simulink model "qss_hybrid_electric_vehicle_example"  (R2023b)
settings: Solver=VariableStepDiscrete  StartTime=0.0  StopTime=1220  RelTol=1e-3  EnableMultiTasking=on
undefined symbols (not defined in the file or in its folder): c_BT_E1, c_BT_E2, c_BT_E3, c_BT_E4, c_BT_L1, c_BT_L2, c_BT_L3, c_BT_L4, h, H_u, I_BT_max, Q_BT_0, Q_BT_IC, rho_f
libraries: qss_tb_library x5
settings Model: Creator=d_goerges  LastModifiedBy=PRATIK
settings SolverCC: AlgebraicLoopSolver=TrustRegion
settings DataIOCC: LimitDataPoints=on  SaveFormat=Array  SignalLoggingSaveFormat=ModelDataLogs  ReturnWorkspaceOutputs=off
settings OptimizationCC: ExpressionDepthLimit=2147483647  LifeSpan=inf
settings DebuggingCC: UnderspecifiedInitializationDetection=Classic  MergeDetectMultiDrivingBlocksExec=none  SolverPrmCheckMsg=warning  FcnCallInpInsideContextMsg=warning  UnconnectedInputMsg=warning  UnconnectedOutputMsg=warning  UnconnectedLineMsg=warning  StateNameClashWarn=warning  SFUnexpectedBacktrackingDiag=warning  SFNoUnconditionalDefaultTransitionDiag=warning  SFExecutionAtInitializationDiag=none  ArithmeticOperatorsInVariantConditions=warning
settings HardwareCC: ProdBitPerPointer=32  ProdBitPerSizeT=32  ProdBitPerPtrDiffT=32  ProdLargestAtomicFloat=None  ProdIntDivRoundTo=Undefined  ProdEndianess=Unspecified  ProdWordSize=32  ProdHWDeviceType=32-bit Generic
settings ModelReferenceCC: PropagateSignalLabelsOutOfModel=off
settings SFSimCC: SimUseLocalCustomCode=off  CustomCodeUndefinedFunction=UseInterfaceOnly
settings RTWCC: RTWUseLocalCustomCode=off
settings CodeAppCC: StateflowObjectComments=on
settings GRTTargetCC: TargetLangStandard=C89/C90 (ANSI)  CombineOutputUpdateFcns=off  GRTInterface=on
settings ConfigComp: CovMetricSettings=dw  CovSaveCumulativeToWorkspaceVar=on  CovSaveSingleToWorkspaceVar=on  CovExternalEMLEnable=off

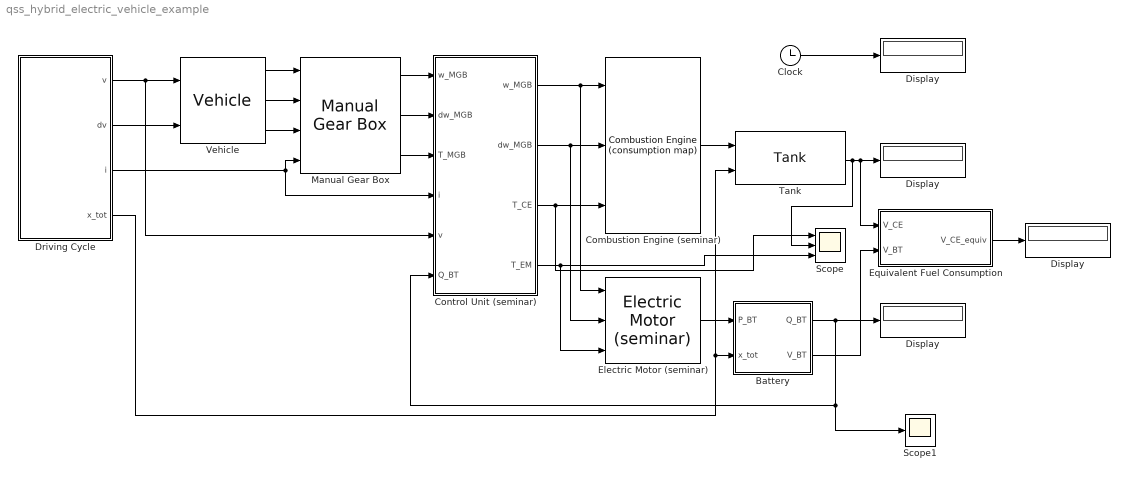
== system qss_hybrid_electric_vehicle_example ==
  "   Display   " : Display
  "  Display  " : Display
  " Display " : Display
  Battery : Subsystem  Tag=battery  AncestorBlock=qss_tb_library/Energy Buffer/Battery  mask(Battery){I_0=10, Q_BT_IC_rel=50, t_ch=2}
      mask prompts: I_0 "Energy capacity of battery [Ah]"; Q_BT_IC_rel "Initial charge of battery [%]"; t_ch "Current limit: minimum time to charge/discharge the battery [min]"
      mask help:
      | This block simulates a battery.
      | The resistance depends on the charge state and the charge/discharge current of the battery. The battery has an open circuit voltage of 130 V (fully charged).
      |
      | Input:
      | =====
      | 	x_tot	Total distance [m]
      | 	P_BT	Power from/to the battery [W]
      | 		P_BT < 0: battery charging
      | 		P_BT > 0: battery discharging
      |
      | Output:
      | ======
      | 	Q_BT	Current charge of the battery [C]
      | 	V_BT	Energy consumption [kWh/100 km]
      mask init:
      | init_BT;
      settings: LibrarySourceBlock=qss_tb_library/Energy Buffer/Battery
  Clock : Clock
  Combustion Engine (seminar) : qss_tb_library/Energy Converter/Combustion Engine (consumption map)  Tag=combustion engine  theta_CE=0.2  w_CE_idle=105  P_CE_idle=8000  P_aux=0  ENABLE_FUEL_CUTOFF=on  T_CE_cutoff=5  P_CE_cutoff=0
  Control Unit (seminar) : Subsystem  Tag=control unit  mask(Control Unit){}
      mask help:
      | This block gives the user the opportunity to design his/her own control unit.
      |
      | The user can define the inputs and outputs  by himself/herself.
      mask init:
      | %init_control_unit;
  Display : Display
  Driving Cycle : Subsystem  Tag=cycle  AncestorBlock=qss_tb_library/Driving Cycle/Driving Cycle  mask(Driving Cycle){cyclenr=Europe: NEDC, stepsize=1, autostop=on}
      mask prompts: cyclenr "Choose a cycle"; stepsize "Step size [s]"; autostop "Enable automatic simulation stop"
      mask help:
      | This block loads the cycle data such as time, speed, acceleration and gear number,  from the specified data file and makes it available on the output of the cycle block.
      |
      | Output:
      | ======
      | 	v	Speed [m/s]
      | 	dv	Acceleration [m/s^2]
      | 	i	Gear number [-]
      | 	x_tot	Total distance [m]
      |
      | Tip:
      | ===
      | Probably you don't need the gear number "i". If so you can terminate
      | it with a "Terminator" out of the "Simulink Library/Connections."
      |
      | Step size:
      | ========
      | Default value is 1. Don't change it, unless you are familiar with the programs of the QSS TB.
      |
      | Enable automatic simulation stop:
      | ===========================
      | Stops the simulation automatically at the end of the cycle.
      | Be careful: If you have a component in your model that has to run after the cycle has finished, e.g. a battery to charge, remove the mark!
      mask init:
      | init_driving_cycle;
      settings: LibrarySourceBlock=qss_tb_library/Driving Cycle/Driving Cycle
      mask TypeOptions cyclenr: Europe: ECE manual | Europe: ECE R15 spez | Europe: ECE R15 | Europe: EUDC | Europe: EUDC manual | Europe: City | Europe: City manual | Europe: NEDC | Europe: NEDC manual | Japan:  10-15-Mode | Japan:  10-Mode | Japan:  10-Mode-3 | Japan:  11-Mode | Japan:  11-Mode-4 | Japan:  15-Mode | USA:    City-I | USA:    City-II | USA:    FTP-75 | USA:    FTP-Highway | Int'l:     WLTC Class 3
      mask Display: plot(T_zplot, V_zplot);
  Electric Motor (seminar) : qss_tb_library/Energy Converter/Electric Motor (seminar)  theta_EM=0.1  P_aux=0
  Equivalent Fuel Consumption : Subsystem  mask(Equivalent Fuel Consumption){eta_BT=0.9, eta_EM=0.8, eta_CE=0.25}
      mask prompts: eta_BT "Battery efficiency [-]"; eta_EM "Motor efficiency [-]"; eta_CE "Engine efficiency [-]"
      mask help:
      | This block computes the equivalent fuel consumption.
      |
      | Input:
      | =====
      | 	V_CE    Fuel consumption [l/100 km]
      | 	V_BT    Energy consumption [kWh/100 km]
      |
      | Output:
      | ======
      | 	V_CE_equiv	Equivalent fuel consumption [l/100 km]
      mask init:
      | init_equivalent_fuel_consumption;
  Manual Gear Box : qss_tb_library/Gear System/Manual Gear Box  Tag=transmission  i_1=3.27  i_2=1.92  i_3=1.26  i_4=0.88  i_5=0.7  i_diff=3.29  e_GT=0.98  P_GT0=100  w_wheel_min=1
  Scope : Scope  NumInputPorts=3
  Scope1 : Scope
  Tank : qss_tb_library/Energy Source/Tank  Tag=tank  fuel=Diesel  flag_cold_start=on
  Vehicle : qss_tb_library/Vehicle/Vehicle  Tag=vehicle  m_f=1115  mt2m_f=5  A_f=2.3  d_wheel=0.576  cw=0.31  mu=0.013
  wires:
  Tank/1 -> Scope/2, Display/1, Equivalent Fuel Consumption/1(V_CE)
  Driving Cycle/2(dv) -> Vehicle/2
  Driving Cycle/1(v) -> Vehicle/1, Control Unit (seminar)/5(v)
  Vehicle/1 -> Manual Gear Box/1
  Vehicle/2 -> Manual Gear Box/2
  Vehicle/3 -> Manual Gear Box/3
  Manual Gear Box/1 -> Control Unit (seminar)/1(w_MGB)
  Manual Gear Box/2 -> Control Unit (seminar)/2(dw_MGB)
  Manual Gear Box/3 -> Control Unit (seminar)/3(T_MGB)
  Control Unit (seminar)/1(" w_MGB ") -> Combustion Engine (seminar)/1, Electric Motor (seminar)/1
  Control Unit (seminar)/2(" dw_MGB ") -> Combustion Engine (seminar)/2, Electric Motor (seminar)/2
  Control Unit (seminar)/3(T_CE) -> Scope/1, Combustion Engine (seminar)/3
  Control Unit (seminar)/4(T_EM) -> Scope/3, Electric Motor (seminar)/3
  Combustion Engine (seminar)/1 -> Tank/1
  Electric Motor (seminar)/1 -> Battery/1(P_BT)
  Driving Cycle/4(x_tot) -> Battery/2(x_tot), Tank/2
  Battery/1(Q_BT) -> "  Display  "/1, Scope1/1, Control Unit (seminar)/6(Q_BT)
  Driving Cycle/3(i) -> Manual Gear Box/4, Control Unit (seminar)/4(i)
  Battery/2(V_BT) -> Equivalent Fuel Consumption/2(V_BT)
  Clock/1 -> " Display "/1
  Equivalent Fuel Consumption/1(V_CE_equiv) -> "   Display   "/1

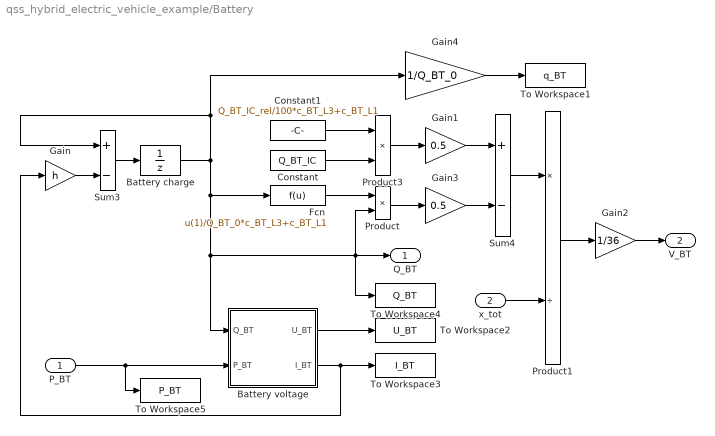
== system qss_hybrid_electric_vehicle_example/Battery ==
  P_BT : Inport
  x_tot : Inport  Port=2
  Battery charge : UnitDelay  InitialCondition=Q_BT_IC  SampleTime=h  HasFrameUpgradeWarning=on
  Battery voltage : Subsystem
  Constant : Constant  Value=Q_BT_IC
  Constant1 : Constant  Value=Q_BT_IC_rel/100*c_BT_L3+c_BT_L1
  Fcn : Fcn  Expr=u(1)/Q_BT_0*c_BT_L3+c_BT_L1
  Gain : Gain  Gain=h  SaturateOnIntegerOverflow=on  OutDataTypeStr=Inherit: Same as input  ParamDataTypeStr=Inherit: Same as input
  Gain1 : Gain  Gain=0.5  SaturateOnIntegerOverflow=on  OutDataTypeStr=Inherit: Same as input  ParamDataTypeStr=Inherit: Same as input
  Gain2 : Gain  Gain=1/36  SaturateOnIntegerOverflow=on  OutDataTypeStr=Inherit: Same as input  ParamDataTypeStr=Inherit: Same as input
  Gain3 : Gain  Gain=0.5  SaturateOnIntegerOverflow=on  OutDataTypeStr=Inherit: Same as input  ParamDataTypeStr=Inherit: Same as input
  Gain4 : Gain  Gain=1/Q_BT_0  SaturateOnIntegerOverflow=on  OutDataTypeStr=Inherit: Same as input  ParamDataTypeStr=Inherit: Same as input
  Product : Product  RndMeth=Zero
  Product1 : Product  Inputs=*/  InputSameDT=on  RndMeth=Zero  SaturateOnIntegerOverflow=on  OutDataTypeStr=Inherit: Same as first input
  Product3 : Product  RndMeth=Zero
  Sum3 : Sum  Inputs=+-  InputSameDT=on  SaturateOnIntegerOverflow=on  OutDataTypeStr=Inherit: Same as first input
  Sum4 : Sum  Inputs=+-  InputSameDT=on  SaturateOnIntegerOverflow=on  OutDataTypeStr=Inherit: Same as first input
  To Workspace1 : ToWorkspace  VariableName=q_BT  SampleTime=-1
  To Workspace2 : ToWorkspace  VariableName=U_BT  SampleTime=-1
  To Workspace3 : ToWorkspace  VariableName=I_BT  SampleTime=-1
  To Workspace4 : ToWorkspace  VariableName=Q_BT  SampleTime=-1
  To Workspace5 : ToWorkspace  VariableName=P_BT  SampleTime=-1
  Q_BT : Outport  InitialOutput=0
  V_BT : Outport  Port=2  InitialOutput=0
  wires:
  Fcn/1 -> Product/1
  Constant1/1 -> Product3/1
  Constant/1 -> Product3/2
  Gain2/1 -> V_BT/1
  Sum4/1 -> Product1/1
  Gain3/1 -> Sum4/2
  Gain1/1 -> Sum4/1
  Product/1 -> Gain3/1
  Product3/1 -> Gain1/1
  P_BT/1 -> To Workspace5/1, Battery voltage/2(P_BT)
  Gain4/1 -> To Workspace1/1
  Product1/1 -> Gain2/1
  x_tot/1 -> Product1/2
  Battery voltage/1(U_BT) -> To Workspace2/1
  Battery charge/1 -> Fcn/1, To Workspace4/1, Q_BT/1, Product/2, Battery voltage/1(Q_BT), Gain4/1, Sum3/1
  Gain/1 -> Sum3/2
  Sum3/1 -> Battery charge/1
  Battery voltage/2(I_BT) -> To Workspace3/1, Gain/1

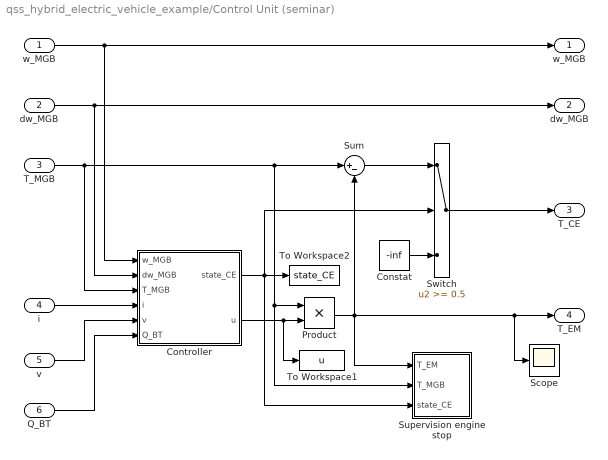
== system qss_hybrid_electric_vehicle_example/Control Unit (seminar) ==
  w_MGB : Inport
  dw_MGB : Inport  Port=2
  T_MGB : Inport  Port=3
  i : Inport  Port=4
  v : Inport  Port=5
  Q_BT : Inport  Port=6
  Constat : Constant  Value=-inf
  Controller : Subsystem  TreatAsAtomicUnit=on
  Product : Product  RndMeth=Zero
  Scope : Scope
  Sum : Sum  Inputs=|+-
  Supervision engine stop : Subsystem
  Switch : Switch  Threshold=0.5  SaturateOnIntegerOverflow=off  InputSameDT=off
  To Workspace1 : ToWorkspace  VariableName=u  SampleTime=-1
  To Workspace2 : ToWorkspace  VariableName=state_CE  SampleTime=-1
  " w_MGB " : Outport  InitialOutput=0
  " dw_MGB " : Outport  Port=2  InitialOutput=0
  T_CE : Outport  Port=3  InitialOutput=0
  T_EM : Outport  Port=4  InitialOutput=0
  wires:
  dw_MGB/1 -> Controller/2(dw_MGB), " dw_MGB "/1
  w_MGB/1 -> Controller/1(w_MGB), " w_MGB "/1
  T_MGB/1 -> Controller/3(T_MGB), Sum/1, Product/1, Supervision engine stop/2(T_MGB)
  Product/1 -> Sum/2, Scope/1, T_EM/1, Supervision engine stop/1(T_EM)
  Controller/2(u) -> To Workspace1/1, Product/2
  i/1 -> Controller/4(i)
  Controller/1(state_CE) -> Switch/2, To Workspace2/1, Supervision engine stop/3(state_CE)
  Sum/1 -> Switch/1
  Switch/1 -> T_CE/1
  Constat/1 -> Switch/3
  v/1 -> Controller/5(v)
  Q_BT/1 -> Controller/6(Q_BT)

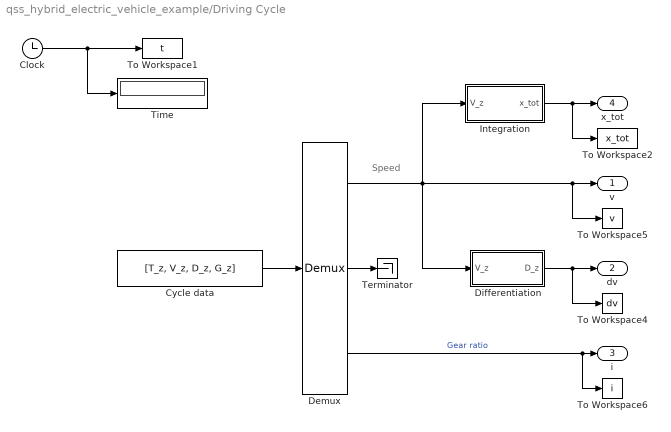
== system qss_hybrid_electric_vehicle_example/Driving Cycle ==
  note: Speed
  Clock : Clock
  Cycle data : FromWorkspace  VariableName=[T_z, V_z, D_z, G_z]  SampleTime=h  ZeroCross=off
  Demux : Demux  Outputs=3
      settings: DisplayOption=none
  Differentiation : Subsystem
  Integration : Subsystem
  Terminator : Terminator
  Time : Display
  To Workspace1 : ToWorkspace  VariableName=t  SampleTime=-1
  To Workspace2 : ToWorkspace  VariableName=x_tot  SampleTime=-1
  To Workspace4 : ToWorkspace  VariableName=dv  SampleTime=-1
  To Workspace5 : ToWorkspace  VariableName=v  SampleTime=-1
  To Workspace6 : ToWorkspace  VariableName=i  SampleTime=-1
  v : Outport  InitialOutput=0
  dv : Outport  Port=2  InitialOutput=0
  i : Outport  Port=3  InitialOutput=0
  x_tot : Outport  Port=4  InitialOutput=0
  wires:
  Clock/1 -> To Workspace1/1, Time/1
  Demux/3 -> To Workspace6/1, i/1  "Gear ratio"
  Integration/1(x_tot) -> To Workspace2/1, x_tot/1
  Demux/1 -> Differentiation/1(V_z), To Workspace5/1, v/1, Integration/1(V_z)
  Demux/2 -> Terminator/1
  Differentiation/1(D_z) -> dv/1, To Workspace4/1
  Cycle data/1 -> Demux/1

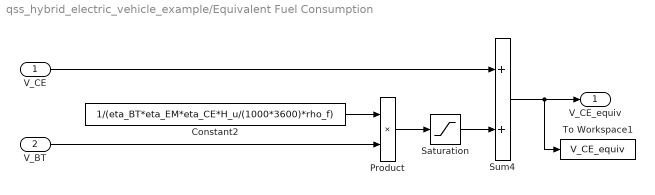
== system qss_hybrid_electric_vehicle_example/Equivalent Fuel Consumption ==
  V_CE : Inport
  V_BT : Inport  Port=2
  Constant2 : Constant  Value=1/(eta_BT*eta_EM*eta_CE*H_u/(1000*3600)*rho_f)
  Product : Product  RndMeth=Zero
  Saturation : Saturate  UpperLimit=inf  LowerLimit=0
  Sum4 : Sum  InputSameDT=on  SaturateOnIntegerOverflow=on  OutDataTypeStr=Inherit: Same as first input
  To Workspace1 : ToWorkspace  VariableName=V_CE_equiv  SampleTime=-1
  V_CE_equiv : Outport
  wires:
  Product/1 -> Saturation/1
  V_BT/1 -> Product/2
  Constant2/1 -> Product/1
  Sum4/1 -> To Workspace1/1, V_CE_equiv/1
  V_CE/1 -> Sum4/1
  Saturation/1 -> Sum4/2

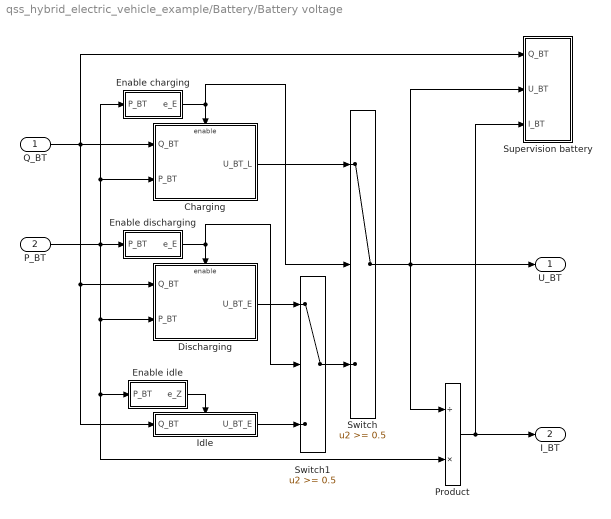
== system qss_hybrid_electric_vehicle_example/Battery/Battery voltage ==
  Q_BT : Inport
  P_BT : Inport  Port=2
  Charging : Subsystem
  Discharging : Subsystem
  Enable charging : Subsystem
  Enable discharging : Subsystem
  Enable idle : Subsystem
  Idle : Subsystem
  Product : Product  Inputs=/*  InputSameDT=on  RndMeth=Zero  SaturateOnIntegerOverflow=on  OutDataTypeStr=Inherit: Same as first input
  Supervision battery : Subsystem
  Switch : Switch  Threshold=0.5
  Switch1 : Switch  Threshold=0.5
  U_BT : Outport  InitialOutput=0
  I_BT : Outport  Port=2  InitialOutput=0
  wires:
  Switch/1 -> U_BT/1, Supervision battery/2(U_BT), Product/1
  Enable charging/1(e_E) -> Switch/2, Charging/Enable
  Q_BT/1 -> Idle/1(Q_BT), Discharging/1(Q_BT), Charging/1(Q_BT), Supervision battery/1(Q_BT)
  Product/1 -> I_BT/1, Supervision battery/3(I_BT)
  Enable discharging/1(e_E) -> Switch1/2, Discharging/Enable
  P_BT/1 -> Enable discharging/1(P_BT), Discharging/2(P_BT), Product/2, Enable idle/1(P_BT), Enable charging/1(P_BT), Charging/2(P_BT)
  Discharging/1(U_BT_E) -> Switch1/1
  Idle/1(U_BT_E) -> Switch1/3
  Switch1/1 -> Switch/3
  Charging/1(U_BT_L) -> Switch/1
  Enable idle/1(e_Z) -> Idle/Enable

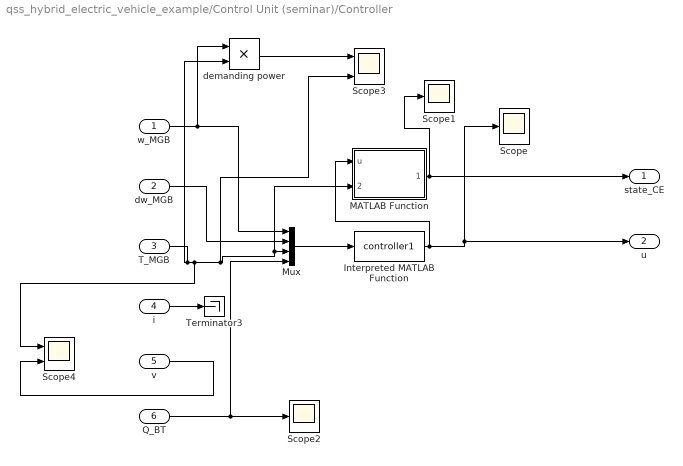
== system qss_hybrid_electric_vehicle_example/Control Unit (seminar)/Controller ==
  w_MGB : Inport
  dw_MGB : Inport  Port=2
  T_MGB : Inport  Port=3
  i : Inport  Port=4
  v : Inport  Port=5
  Q_BT : Inport  Port=6
  Interpreted MATLAB Function : MATLABFcn  MATLABFcn=controller1
  MATLAB Function : MATLAB Function  TreatAsAtomicUnit=on
  Mux : Mux
  Scope : Scope
  Scope1 : Scope
  Scope2 : Scope
  Scope3 : Scope  NumInputPorts=2
  Scope4 : Scope  NumInputPorts=2
  Terminator3 : Terminator
  demanding power : Product
  state_CE : Outport  InitialOutput=0
  u : Outport  Port=2  InitialOutput=0
  wires:
  i/1 -> Terminator3/1
  v/1 -> Scope4/2
  w_MGB/1 -> demanding power/1, Mux/1
  dw_MGB/1 -> Mux/2
  T_MGB/1 -> Scope3/2, MATLAB Function/2(T_MGB), Mux/3, Scope4/1, demanding power/2
  Mux/1 -> Interpreted MATLAB Function/1
  Interpreted MATLAB Function/1 -> MATLAB Function/1(u), u/1, Scope/1
  Q_BT/1 -> Mux/4, Scope2/1
  demanding power/1 -> Scope3/1
  MATLAB Function/1(CE_STATE) -> Scope1/1, state_CE/1

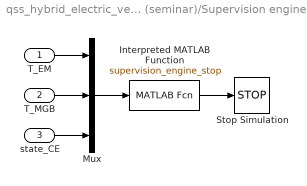
== system qss_hybrid_electric_vehicle_example/Control Unit (seminar)/Supervision engine stop ==
  T_EM : Inport
  T_MGB : Inport  Port=2
  state_CE : Inport  Port=3
  Interpreted MATLAB Function : MATLABFcn  MATLABFcn=supervision_engine_stop
  Mux : Mux  Inputs=3
  Stop Simulation : Stop
  wires:
  T_MGB/1 -> Mux/2
  T_EM/1 -> Mux/1
  state_CE/1 -> Mux/3
  Mux/1 -> Interpreted MATLAB Function/1
  Interpreted MATLAB Function/1 -> Stop Simulation/1

== system qss_hybrid_electric_vehicle_example/Driving Cycle/Differentiation ==
  V_z : Inport
  Sum1 : Sum  Inputs=+-  InputSameDT=on  SaturateOnIntegerOverflow=on  OutDataTypeStr=Inherit: Same as first input
  Unit Delay1 : UnitDelay  SampleTime=h  HasFrameUpgradeWarning=on
  D_z : Outport  InitialOutput=0
  wires:
  Sum1/1 -> D_z/1
  V_z/1 -> Unit Delay1/1, Sum1/1
  Unit Delay1/1 -> Sum1/2

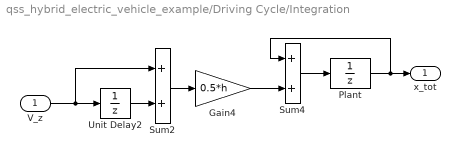
== system qss_hybrid_electric_vehicle_example/Driving Cycle/Integration ==
  V_z : Inport
  Gain4 : Gain  Gain=0.5*h  SaturateOnIntegerOverflow=on  OutDataTypeStr=Inherit: Same as input  ParamDataTypeStr=Inherit: Same as input
  Plant : UnitDelay  InitialCondition=1  SampleTime=h  HasFrameUpgradeWarning=on
  Sum2 : Sum  InputSameDT=on  SaturateOnIntegerOverflow=on  OutDataTypeStr=Inherit: Same as first input
  Sum4 : Sum  InputSameDT=on  SaturateOnIntegerOverflow=on  OutDataTypeStr=Inherit: Same as first input
  Unit Delay2 : UnitDelay  SampleTime=h  HasFrameUpgradeWarning=on
  x_tot : Outport  InitialOutput=0
  wires:
  Plant/1 -> x_tot/1, Sum4/1
  Sum4/1 -> Plant/1
  Gain4/1 -> Sum4/2
  V_z/1 -> Unit Delay2/1, Sum2/1
  Unit Delay2/1 -> Sum2/2
  Sum2/1 -> Gain4/1

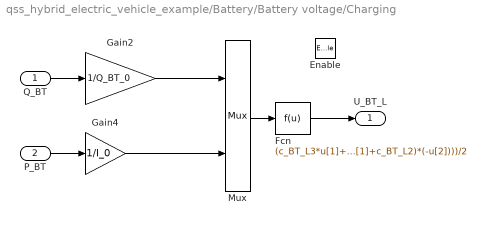
== system qss_hybrid_electric_vehicle_example/Battery/Battery voltage/Charging ==
  Q_BT : Inport
  P_BT : Inport  Port=2
  Enable : EnablePort
  Fcn : Fcn  Expr=(c_BT_L3*u[1]+c_BT_L1+sqrt((c_BT_L3*u[1]+c_BT_L1)^2+4*(c_BT_L4*u[1]+c_BT_L2)*(-u[2])))/2
  Gain2 : Gain  Gain=1/Q_BT_0  SaturateOnIntegerOverflow=on  OutDataTypeStr=Inherit: Same as input  ParamDataTypeStr=Inherit: Same as input
  Gain4 : Gain  Gain=1/I_0  SaturateOnIntegerOverflow=on  OutDataTypeStr=Inherit: Same as input  ParamDataTypeStr=Inherit: Same as input
  Mux : Mux  Inputs=2
  U_BT_L : Outport  InitialOutput=0
  wires:
  Fcn/1 -> U_BT_L/1
  Mux/1 -> Fcn/1
  P_BT/1 -> Gain4/1
  Q_BT/1 -> Gain2/1
  Gain2/1 -> Mux/1
  Gain4/1 -> Mux/2

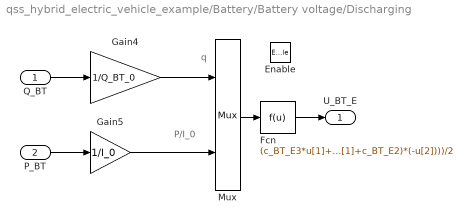
== system qss_hybrid_electric_vehicle_example/Battery/Battery voltage/Discharging ==
  note: P/I_0
  note: q
  Q_BT : Inport
  P_BT : Inport  Port=2
  Enable : EnablePort
  Fcn : Fcn  Expr=(c_BT_E3*u[1]+c_BT_E1+sqrt((c_BT_E3*u[1]+c_BT_E1)^2+4*(c_BT_E4*u[1]+c_BT_E2)*(-u[2])))/2
  Gain4 : Gain  Gain=1/Q_BT_0  SaturateOnIntegerOverflow=on  OutDataTypeStr=Inherit: Same as input  ParamDataTypeStr=Inherit: Same as input
  Gain5 : Gain  Gain=1/I_0  SaturateOnIntegerOverflow=on  OutDataTypeStr=Inherit: Same as input  ParamDataTypeStr=Inherit: Same as input
  Mux : Mux  Inputs=2
  U_BT_E : Outport  InitialOutput=0
  wires:
  Mux/1 -> Fcn/1
  Gain5/1 -> Mux/2
  Gain4/1 -> Mux/1
  P_BT/1 -> Gain5/1
  Q_BT/1 -> Gain4/1
  Fcn/1 -> U_BT_E/1

== system qss_hybrid_electric_vehicle_example/Battery/Battery voltage/Enable charging ==
  P_BT : Inport
  Gain : Gain  Gain=-1  SaturateOnIntegerOverflow=on  OutDataTypeStr=Inherit: Same as input  ParamDataTypeStr=Inherit: Same as input
  Saturation : Saturate  UpperLimit=0  LowerLimit=-inf
  Sign : Signum
  e_E : Outport  InitialOutput=0
  wires:
  Gain/1 -> Sign/1
  Saturation/1 -> Gain/1
  Sign/1 -> e_E/1
  P_BT/1 -> Saturation/1

== system qss_hybrid_electric_vehicle_example/Battery/Battery voltage/Enable discharging ==
  P_BT : Inport
  Saturation : Saturate  UpperLimit=inf  LowerLimit=0
  Sign : Signum
  e_E : Outport  InitialOutput=0
  wires:
  Saturation/1 -> Sign/1
  Sign/1 -> e_E/1
  P_BT/1 -> Saturation/1

== system qss_hybrid_electric_vehicle_example/Battery/Battery voltage/Enable idle ==
  P_BT : Inport
  Abs : Abs
  Constant : Constant
  Sign : Signum
  Sum4 : Sum  Inputs=-+  InputSameDT=on  SaturateOnIntegerOverflow=on  OutDataTypeStr=Inherit: Same as first input
  e_Z : Outport  InitialOutput=0
  wires:
  Constant/1 -> Sum4/2
  Sum4/1 -> e_Z/1
  Abs/1 -> Sum4/1
  Sign/1 -> Abs/1
  P_BT/1 -> Sign/1

== system qss_hybrid_electric_vehicle_example/Battery/Battery voltage/Idle ==
  Q_BT : Inport
  Enable : EnablePort  StatesWhenEnabling=reset
  Constant : Constant  Value=c_BT_L1
  Gain4 : Gain  Gain=c_BT_L3/Q_BT_0  SaturateOnIntegerOverflow=on  OutDataTypeStr=Inherit: Same as input  ParamDataTypeStr=Inherit: Same as input
  Sum8 : Sum  InputSameDT=on  SaturateOnIntegerOverflow=on  OutDataTypeStr=Inherit: Same as first input
  U_BT_E : Outport  InitialOutput=0
  wires:
  Sum8/1 -> U_BT_E/1
  Constant/1 -> Sum8/2
  Gain4/1 -> Sum8/1
  Q_BT/1 -> Gain4/1

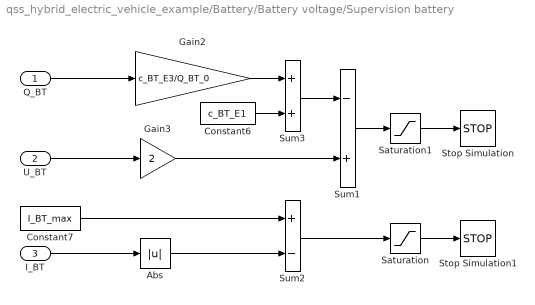
== system qss_hybrid_electric_vehicle_example/Battery/Battery voltage/Supervision battery ==
  Q_BT : Inport
  U_BT : Inport  Port=2
  I_BT : Inport  Port=3
  Abs : Abs
  Constant6 : Constant  Value=c_BT_E1
  Constant7 : Constant  Value=I_BT_max
  Gain2 : Gain  Gain=c_BT_E3/Q_BT_0  SaturateOnIntegerOverflow=on  OutDataTypeStr=Inherit: Same as input  ParamDataTypeStr=Inherit: Same as input
  Gain3 : Gain  Gain=2  SaturateOnIntegerOverflow=on  OutDataTypeStr=Inherit: Same as input  ParamDataTypeStr=Inherit: Same as input
  Saturation : Saturate  UpperLimit=0  LowerLimit=-inf
  Saturation1 : Saturate  UpperLimit=0  LowerLimit=-inf
  Stop Simulation : Stop
  Stop Simulation1 : Stop
  Sum1 : Sum  Inputs=-+  InputSameDT=on  SaturateOnIntegerOverflow=on  OutDataTypeStr=Inherit: Same as first input
  Sum2 : Sum  Inputs=+-  InputSameDT=on  SaturateOnIntegerOverflow=on  OutDataTypeStr=Inherit: Same as first input
  Sum3 : Sum  InputSameDT=on  SaturateOnIntegerOverflow=on  OutDataTypeStr=Inherit: Same as first input
  wires:
  Q_BT/1 -> Gain2/1
  Abs/1 -> Sum2/2
  I_BT/1 -> Abs/1
  Sum2/1 -> Saturation/1
  Constant7/1 -> Sum2/1
  Gain2/1 -> Sum3/1
  Constant6/1 -> Sum3/2
  Sum1/1 -> Saturation1/1
  Saturation1/1 -> Stop Simulation/1
  Gain3/1 -> Sum1/2
  U_BT/1 -> Gain3/1
  Sum3/1 -> Sum1/1
  Saturation/1 -> Stop Simulation1/1

== matlab function qss_hybrid_electric_vehicle_example/Control Unit (seminar)/Controller/MATLAB Function ==
  data: u input; CE_STATE output; T_MGB input
function CE_STATE = fcn(u,T_MGB)
if (T_MGB<0 && u==1) || (T_MGB>0 && u==1) || T_MGB == 0
    CE_STATE=0;
else 
    CE_STATE=1;



end
